simulink model "Full_Integration_with_sensor_redudancy"  (R2024b)
settings: Solver=VariableStepAuto  StartTime=0.0  StopTime=500  RelTol=1e-3
undefined symbols (not defined in the file): Bm1, Bm2, Br, Bsc, Btr, Continuous, G, Im1, Im2, Isw, Jtr, Ke, Ke2, kp, kr, ks, Ksc, Ksr, Kt, Kt2, ktr, Kv1, Kv2, L1, L2, lf, lr, Mr, N, n, n1, R1, R2, rp, Tfrc, Time, to, Vx
libraries: simulink_extras x3, simulink x2, slpidlib x1, ctrlSharedLib x1
settings Model: Creator=Timothy  LastModifiedBy=HP
settings OptimizationCC: ReuseModelBlockBuffer=off
settings RTWCC: GPUComputeCapability=3.5

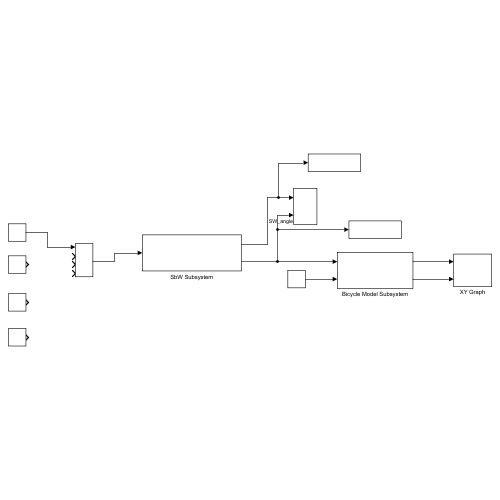
[thumbnail: Simulink's stored preview of the top-level diagram]
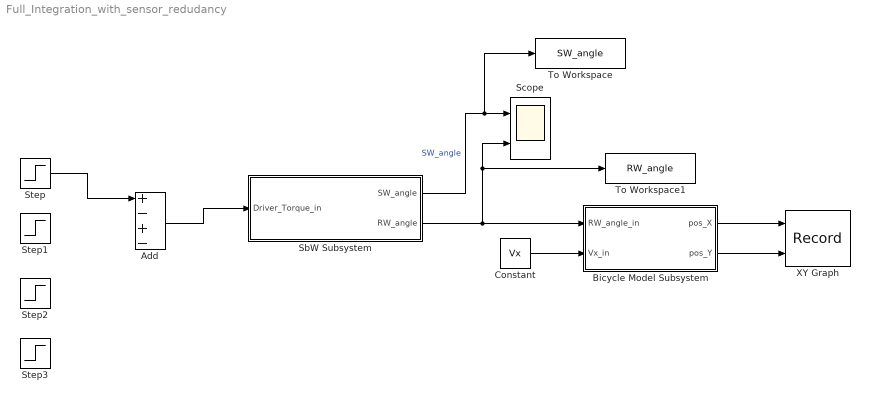
== system Full_Integration_with_sensor_redudancy ==
  Add : Sum  Inputs=+-+-
  Bicycle Model Subsystem : Subsystem
  Constant : Constant  Value=Vx
  SbW Subsystem : Subsystem
  Scope : Scope  NumInputPorts=2
  Step : Step  Time=0  After=0.5  SampleTime=0
  Step1 : Step  Time=30.1  After=0.5  SampleTime=0
  Step2 : Step  Time=60  After=-0.5  SampleTime=0
  Step3 : Step  Time=60.1  After=-0.5  SampleTime=0
  To Workspace : ToWorkspace  VariableName=SW_angle  SaveFormat=Timeseries  SampleTime=-1
  To Workspace1 : ToWorkspace  VariableName=RW_angle  SaveFormat=Timeseries  SampleTime=-1
  XY Graph : Record  FileSettingsInternal="{\"entries\":[{\"content\":{\"excelSettings\":{\"content\":{},\"type\":\"Streamout.ExcelSettings\"}},\"type\":\"Streamout.FileSettingStorage\",\"uuid\":\"\"}],\"packageUris\":[\"http:\\/\\/schema.mathworks.com\\/mf0\\/streamout_blocks\\/R2020a\"],\"version\":\"1.0\"}"  Layout=[1 1]  SignalsInternal="{\"entries\":[{\"content\":{\"signals\":[{\"content\":{\"blockPath\":[],\"dimensions\":[1],\"domain\":\"\",\"lineColor\":\"#a2142f\",\"plots\":[ 1 ],\"port\":1,\"sid\":[\"\"],\"signalID\":1,\"signalName\":\"Bicycle Model Subsystem:1\"},\"type\":\"RecordBlkView.Signal\",\"uuid\":\"\"},{\"content\":{\"blockPath\":[],\"dimensions\":[1],\"domain\":\"\",\"lineColor\":\"#139fff\",\"plots\":[ 1 ],\"port\":2,\"sid\":[\"\"],\"signalID\":2,\"signalName\":\"Bicycle Model Subsystem:2\"},\"type\":\"RecordBlkView.Signal\",\"uuid\":\"\"}]},\"type\":\"RecordBlkView.InputSignals\",\"uuid\":\"\"}],\"packageUris\":[\"http:\\/\\/schema.mathworks.com\\/mf0\\/streamout_blocks\\/R2020a\"],\"version\":\"1.0\"}"  VisualizationBindings="{\"xyplotplugin\":{\"info\":[{\"series\":[{\"bindingParametersList\":[{\"parameter\":\"X-Axis\",\"signalID\":1,\"signalName\":\"Bicycle Model Subsystem:1\"},{\"parameter\":\"Y-Axis\",\"signalID\":2,\"signalName\":\"Bicycle Model Subsystem:2\"}],\"seriesID\":0}],\"subplotID\":1}]}}"  CompatibilityTag=XY
  wires:
  SbW Subsystem/2(RW_angle) -> To Workspace1/1, Scope/2, Bicycle Model Subsystem/1(RW_angle_in)
  SbW Subsystem/1(SW_angle) -> To Workspace/1, Scope/1  "SW_angle"
  Constant/1 -> Bicycle Model Subsystem/2(Vx_in)
  Add/1 -> SbW Subsystem/1(Driver_Torque_in)
  Bicycle Model Subsystem/1(pos_X) -> XY Graph/1
  Bicycle Model Subsystem/2(pos_Y) -> XY Graph/2
  Step/1 -> Add/1

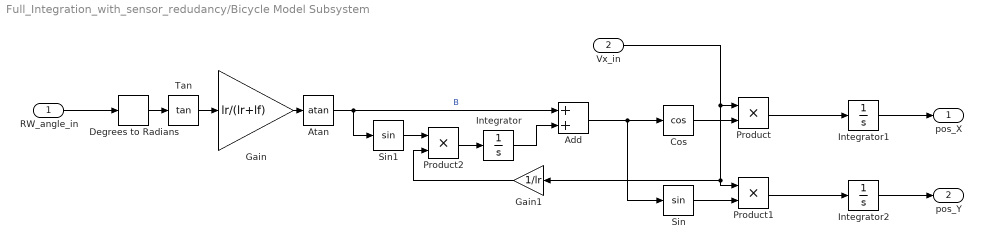
== system Full_Integration_with_sensor_redudancy/Bicycle Model Subsystem ==
  RW_angle_in : Inport
  Vx_in : Inport  Port=2
  Add : Sum
  Atan : Trigonometry  Operator=atan
  Cos : Trigonometry  Operator=cos
  Degrees to Radians : simulink_extras/Transformations/Degrees to Radians
  Gain : Gain  Gain=lr/(lr+lf)
  Gain1 : Gain  Gain=1/lr
  Integrator : Integrator
  Integrator1 : Integrator
  Integrator2 : Integrator
  Product : Product
  Product1 : Product
  Product2 : Product
  Sin : Trigonometry
  Sin1 : Trigonometry
  Tan : Trigonometry  Operator=tan
  pos_X : Outport
  pos_Y : Outport  Port=2
  wires:
  Degrees to Radians/1 -> Tan/1
  Product2/1 -> Integrator/1
  Cos/1 -> Product/2
  Add/1 -> Sin/1, Cos/1
  Atan/1 -> Add/1, Sin1/1  "B"
  Vx_in/1 -> Product1/1, Gain1/1, Product/1
  Integrator1/1 -> pos_X/1
  Gain1/1 -> Product2/2
  Integrator/1 -> Add/2
  Integrator2/1 -> pos_Y/1
  Gain/1 -> Atan/1
  Product/1 -> Integrator1/1
  Product1/1 -> Integrator2/1
  Tan/1 -> Gain/1
  RW_angle_in/1 -> Degrees to Radians/1
  Sin1/1 -> Product2/1
  Sin/1 -> Product1/2

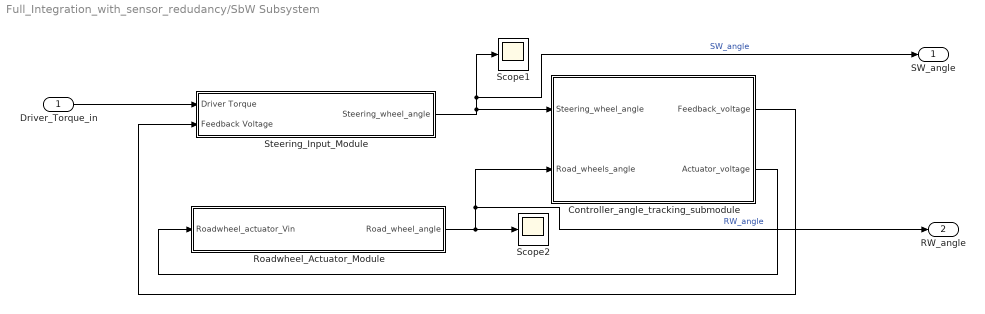
== system Full_Integration_with_sensor_redudancy/SbW Subsystem ==
  Driver_Torque_in : Inport
  Controller_angle_tracking_submodule : Subsystem
  Roadwheel_Actuator_Module : Subsystem
  Scope1 : Scope
  Scope2 : Scope
  Steering_Input_Module : Subsystem
  SW_angle : Outport
  RW_angle : Outport  Port=2
  wires:
  Roadwheel_Actuator_Module/1(Road_wheel_angle) -> Scope2/1, RW_angle/1, Controller_angle_tracking_submodule/2(Road_wheels_angle)  "RW_angle"
  Steering_Input_Module/1(Steering_wheel_angle) -> SW_angle/1, Scope1/1, Controller_angle_tracking_submodule/1(Steering_wheel_angle)  "SW_angle"
  Controller_angle_tracking_submodule/2(Actuator_voltage) -> Roadwheel_Actuator_Module/1(Roadwheel_actuator_Vin)
  Driver_Torque_in/1 -> Steering_Input_Module/1(Driver Torque)
  Controller_angle_tracking_submodule/1(Feedback_voltage) -> Steering_Input_Module/2(Feedback Voltage)

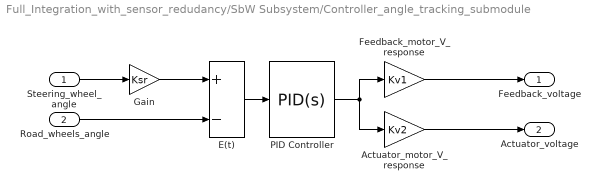
== system Full_Integration_with_sensor_redudancy/SbW Subsystem/Controller_angle_tracking_submodule ==
  Steering_wheel_angle : Inport
  Road_wheels_angle : Inport  Port=2
  Actuator_motor_V_response : Gain  Gain=Kv2
  E(t) : Sum  Inputs=+-
  Feedback_motor_V_response : Gain  Gain=Kv1
  Gain : Gain  Gain=Ksr
  PID Controller : slpidlib/PID Controller  Controller=PID  Form=Parallel  TimeDomain=Continuous-time  UseExternalTs=off  SampleTime=-1  IntegratorMethod=Forward Euler  FilterMethod=Forward Euler  ControllerParametersSource=internal  P=20  I=1  UseKiTs=off  D=-0.5  UseExternalDerivativeSource=off  N=100  UseFilter=on  TunerSelectOption=Transfer Function Based (PID Tuner App)  InitialConditionSource=internal  InitialConditionForIntegrator=0  InitialConditionForFilter=0  DifferentiatorICPrevScaledInput=0  ExternalReset=none  TrackingMode=off  Kt=1  LimitOutput=off  SatLimitsSource=internal  UpperSaturationLimit=100  LowerSaturationLimit=-100  LinearizeAsGain=on  AntiWindupMode=none  Kb=1  LimitIntegrator=off  UpperIntegratorSaturationLimit=inf  LowerIntegratorSaturationLimit=-inf  POutMin=[]  POutMax=[]  IOutMin=[]  IOutMax=[]  DOutMin=[]  DOutMax=[]  NOutMin=[]  NOutMax=[]  SumOutMin=[]  SumOutMax=[]  SaturationOutMin=[]  SaturationOutMax=[]  PParamMin=[]  PParamMax=[]  IParamMin=[]  IParamMax=[]  DParamMin=[]  DParamMax=[]  NParamMin=[]  NParamMax=[]  KbParamMin=[]  KbParamMax=[]  KtParamMin=[]  KtParamMax=[]  KbOutMin=[]  KbOutMax=[]  KtOutMin=[]  KtOutMax=[]  IntegratorOutMin=[]  IntegratorOutMax=[]  FilterOutMin=[]  FilterOutMax=[]  SumI1OutMin=[]  SumI1OutMax=[]  SumI2OutMin=[]  SumI2OutMax=[]  SumI3OutMin=[]  SumI3OutMax=[]  SumI4OutMin=[]  SumI4OutMax=[]  SumDOutMin=[]  SumDOutMax=[]  DifferentiatorOutMin=[]  DifferentiatorOutMax=[]  FilterDiffOutCoefMin=[]  FilterDiffOutCoefMax=[]  ReciprocalOutMin=[]  ReciprocalOutMax=[]  SumDenOutMin=[]  SumDenOutMax=[]  SumNumOutMin=[]  SumNumOutMax=[]  DivideOutMin=[]  DivideOutMax=[]  UdiffTsProdOutMin=[]  UdiffTsProdOutMax=[]  NTsProdOutMin=[]  NTsProdOutMax=[]  UintegralTsProdOutMin=[]  UintegralTsProdOutMax=[]  UngainTsProdOutMin=[]  UngainTsProdOutMax=[]  ClampingZeroOutDataTypeStr=Inherit: Inherit via back propagation  ClampingZeroOutMin=[]  ClampingZeroOutMax=[]  FilterDenConstantOutDataTypeStr=Inherit: Inherit via back propagation  FilterDenConstantOutMin=[]  FilterDenConstantOutMax=[]  PCopyOutDataTypeStr=Inherit: Inherit via back propagation  PCopyOutMin=[]  PCopyOutMax=[]  NCopyOutDataTypeStr=Inherit: Inherit via back propagation  NCopyOutMin=[]  NCopyOutMax=[]  IntegratorContinuousStateAttributes=''  IntegratorStateMustResolveToSignalObject=off  IntegratorRTWStateStorageClass=Auto  FilterContinuousStateAttributes=''  FilterStateMustResolveToSignalObject=off  FilterRTWStateStorageClass=Auto  ParallelPVariant=InternalParameters  IdealPVariant=Disabled  IVariant=InternalParameters  DVariant=InternalParameters  IntegratorVariant=Continuous  SatVariant=Disabled  AWVariant=Passthrough  PCopyVariant=Disabled  TRVariant=Disabled  FdbkBlocksVariant=Forward  IdealPFdbkVariant=Disabled  SatFdbkVariant=Disabled  DerivativeFilterVariant=ContFilter  NVariant=InternalParameters  NCopyVariant=Disabled  FilterICVariant=InternalICsFilter  IntegratorICVariant=InternalICs  ExternalResetVariant=Disabled  TRSumVariant=Passthrough  SumFdbkVariant=Disabled  SumVariant=Sum_PID  TsampFilterVariant=InternalTs  TsampNgainVariant=Passthrough  TsampIntegralVariant=Disabled_SignalSpec  ExternalSaturationOutDataTypeStr=Inherit: Same as second input  DerivativeSourceVariant=ErrorSignal  PreIntVariant=InternalPreInt
  Feedback_voltage : Outport
  Actuator_voltage : Outport  Port=2
  wires:
  Feedback_motor_V_response/1 -> Feedback_voltage/1
  E(t)/1 -> PID Controller/1
  PID Controller/1 -> Actuator_motor_V_response/1, Feedback_motor_V_response/1
  Road_wheels_angle/1 -> E(t)/2
  Steering_wheel_angle/1 -> Gain/1
  Actuator_motor_V_response/1 -> Actuator_voltage/1
  Gain/1 -> E(t)/1

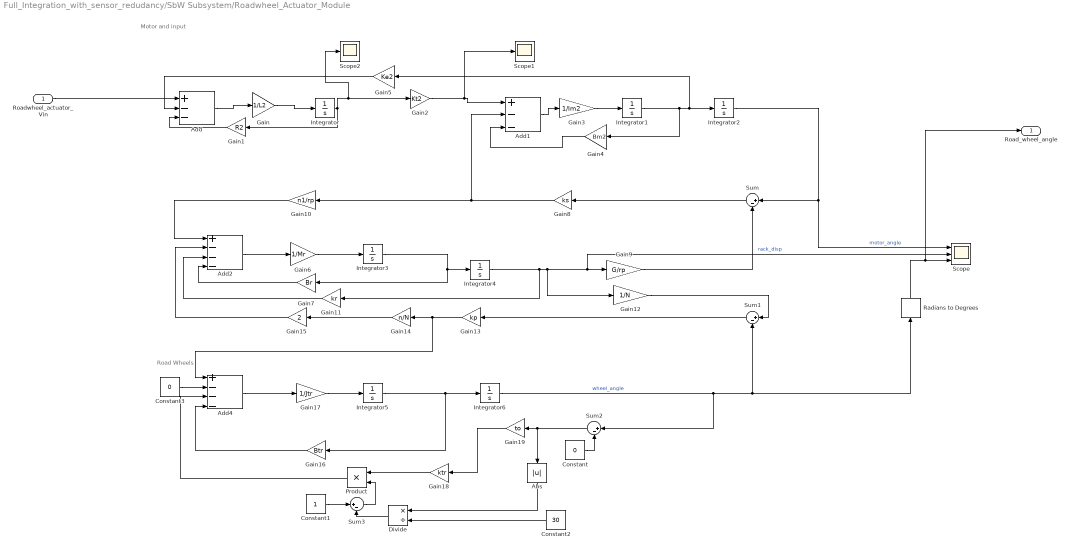
== system Full_Integration_with_sensor_redudancy/SbW Subsystem/Roadwheel_Actuator_Module ==
  note: Road Wheels
  note: Motor and input
  Roadwheel_actuator_Vin : Inport
  Abs : Abs  SaturateOnIntegerOverflow=off
  Add : Sum  Inputs=+--
  Add1 : Sum  Inputs=+--
  Add2 : Sum  Inputs=+---
  Add4 : Sum  Inputs=+---
  Constant : Constant  Value=0
  Constant1 : Constant
  Constant2 : Constant  Value=30
  Constant3 : Constant  Value=0
  Divide : Product  Inputs=*/
  Gain : Gain  Gain=1/L2
  Gain1 : Gain  Gain=R2
  Gain10 : Gain  Gain=n1/rp
  Gain11 : Gain  Gain=kr
  Gain12 : Gain  Gain=1/N
  Gain13 : Gain  Gain=kp
  Gain14 : Gain  Gain=n/N
  Gain15 : Gain  Gain=2
  Gain16 : Gain  Gain=Btr
  Gain17 : Gain  Gain=1/Jtr
  Gain18 : Gain  Gain=ktr
  Gain19 : Gain  Gain=to
  Gain2 : Gain  Gain=Kt2
  Gain3 : Gain  Gain=1/Im2
  Gain4 : Gain  Gain=Bm2
  Gain5 : Gain  Gain=Ke2
  Gain6 : Gain  Gain=1/Mr
  Gain7 : Gain  Gain=Br
  Gain8 : Gain  Gain=ks
  Gain9 : Gain  Gain=G/rp
  Integrator{,1..6} (7 alike) : Integrator
  Product : Product
  Radians to Degrees : simulink_extras/Transformations/Radians to Degrees
  Scope : Scope  NumInputPorts=3
  Scope1 : Scope
  Scope2 : Scope
  Sum{,1..3} (4 alike) : Sum  Inputs=|+-
  Road_wheel_angle : Outport
  wires:
  Gain11/1 -> Add2/3
  Abs/1 -> Divide/1
  Gain5/1 -> Add/2
  Integrator2/1 -> Sum/1, Scope/1  "motor_angle"
  Add1/1 -> Gain3/1
  Gain2/1 -> Scope1/1, Add1/1
  Gain3/1 -> Integrator1/1
  Gain13/1 -> Add4/1, Gain14/1
  Integrator6/1 -> Radians to Degrees/1, Sum1/2, Sum2/1  "wheel_angle"
  Gain6/1 -> Integrator3/1
  Constant1/1 -> Sum3/1
  Roadwheel_actuator_Vin/1 -> Add/1
  Divide/1 -> Sum3/2
  Gain10/1 -> Add2/1
  Integrator/1 -> Gain1/1, Gain2/1, Scope2/1
  Gain1/1 -> Add/3
  Add4/1 -> Gain17/1
  Add/1 -> Gain/1
  Integrator1/1 -> Gain4/1, Gain5/1, Integrator2/1
  Constant2/1 -> Divide/2
  Sum/1 -> Gain8/1
  Sum3/1 -> Product/2
  Gain12/1 -> Sum1/1
  Gain19/1 -> Gain18/1
  Gain15/1 -> Add2/2
  Product/1 -> Add4/3
  Gain18/1 -> Product/1
  Integrator4/1 -> Gain11/1, Gain12/1, Scope/2, Gain9/1  "rack_disp"
  Sum2/1 -> Abs/1, Gain19/1
  Gain9/1 -> Sum/2
  Add2/1 -> Gain6/1
  Integrator3/1 -> Gain7/1, Integrator4/1
  Constant3/1 -> Add4/2
  Gain4/1 -> Add1/3
  Integrator5/1 -> Gain16/1, Integrator6/1
  Gain14/1 -> Gain15/1
  Constant/1 -> Sum2/2
  Sum1/1 -> Gain13/1
  Radians to Degrees/1 -> Road_wheel_angle/1, Scope/3
  Gain16/1 -> Add4/4
  Gain8/1 -> Gain10/1, Add1/2
  Gain17/1 -> Integrator5/1
  Gain/1 -> Integrator/1
  Gain7/1 -> Add2/4

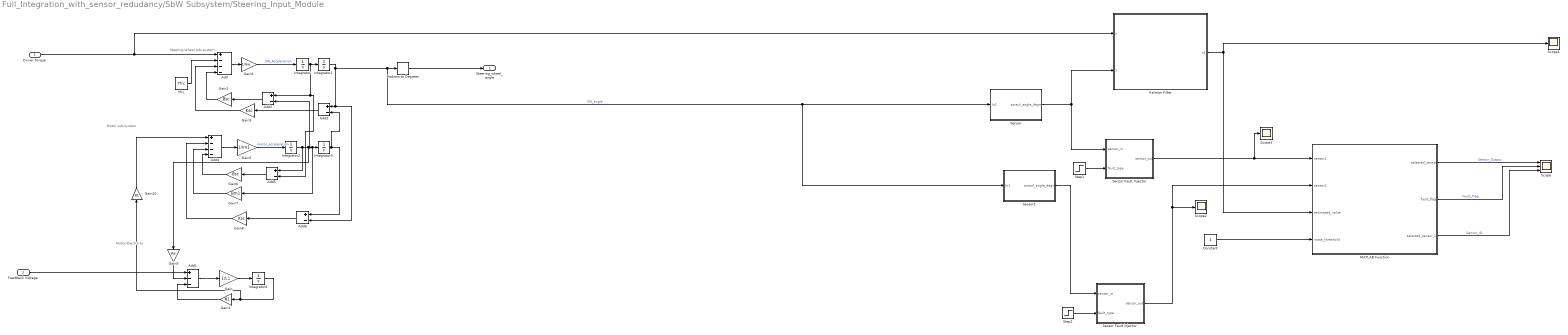
== system Full_Integration_with_sensor_redudancy/SbW Subsystem/Steering_Input_Module ==
  note: Steering Wheel sub-system
  note: Motor-Electrical
  note: Motor sub-system
  Driver Torque : Inport
  Feedback Voltage : Inport  Port=2
  Add : Sum  Inputs=+---
  Add1 : Sum  Inputs=+--
  Add{2..3,5..6} (4 alike) : Sum  Inputs=+-
  Add4 : Sum  Inputs=+---
  Constant : Constant
  Gain : Gain  Gain=1/L1
  Gain1 : Gain  Gain=R1
  Gain10 : Gain  Gain=Kt
  Gain2 : Gain  Gain=Bsc
  Gain3 : Gain  Gain=Ksc
  Gain4 : Gain  Gain=1/Isw
  Gain5 : Gain  Gain=1/Im1
  Gain6 : Gain  Gain=Bsc
  Gain7 : Gain  Gain=Bm1
  Gain8 : Gain  Gain=Ksc
  Gain9 : Gain  Gain=Ke
  Integrator{,1..4} (5 alike) : Integrator
  Kalman Filter : Subsystem
  MATLAB Function : MATLAB Function  TreatAsAtomicUnit=on
  Radians to Degrees : simulink_extras/Transformations/Radians to Degrees
  Scope : Scope  NumInputPorts=3
  Scope1 : Scope
  Scope2 : Scope
  Scope3 : Scope
  Sensor : Subsystem
  Sensor Fault Injector : MATLAB Function  TreatAsAtomicUnit=on
  Sensor Fault injector : MATLAB Function  TreatAsAtomicUnit=on
  Sensor1 : Subsystem
  Step1 : Step  Time=0  SampleTime=0
  Step2 : Step  Time=0  After=2  SampleTime=0
  Tfrc : Constant  Value=Tfrc
  Steering_wheel_angle : Outport
  wires:
  Gain2/1 -> Add/4
  Integrator1/1 -> Add6/2, Add3/1, Sensor1/1(In1), Sensor/1(In1), Radians to Degrees/1  "SW_angle"
  Gain10/1 -> Add4/1
  Gain6/1 -> Add4/4
  Gain8/1 -> Add4/2
  Tfrc/1 -> Add/2
  Gain1/1 -> Add1/3
  Integrator/1 -> Integrator1/1, Add2/1, Add5/2
  Add3/1 -> Gain3/1
  Integrator3/1 -> Add3/2, Add6/1
  Integrator2/1 -> Gain9/1, Add2/2, Gain7/1, Integrator3/1, Add5/1
  Add/1 -> Gain4/1
  Add6/1 -> Gain8/1
  Feedback Voltage/1 -> Add1/1
  Gain/1 -> Integrator4/1
  Gain5/1 -> Integrator2/1  "motor_acceleration"
  Gain7/1 -> Add4/3
  Add1/1 -> Gain/1
  Gain3/1 -> Add/3
  Integrator4/1 -> Gain1/1, Gain10/1
  Add2/1 -> Gain2/1
  Add4/1 -> Gain5/1
  Driver Torque/1 -> Kalman Filter/1(u), Add/1
  Add5/1 -> Gain6/1
  Radians to Degrees/1 -> Steering_wheel_angle/1
  Gain9/1 -> Add1/2
  Gain4/1 -> Integrator/1  "SW_Acceleration"
  Sensor/1(actaul_angle_degre) -> Sensor Fault Injector/1(sensor_in), Kalman Filter/2(y)
  Constant/1 -> MATLAB Function/4(noise_threshold)
  MATLAB Function/1(selected_sensor) -> Scope/1  "Sensor_Output"
  MATLAB Function/2(fault_flag) -> Scope/2  "Fault_Flag"
  MATLAB Function/3(selected_sensor_id) -> Scope/3  "Sensor_ID"
  Kalman Filter/1(s1) -> MATLAB Function/3(estimated_value), Scope1/1
  Sensor1/1(actaul_angle_degre) -> Sensor Fault injector/1(sensor_in)
  Sensor Fault injector/1(sensor_out) -> MATLAB Function/2(sensor2), Scope2/1
  Sensor Fault Injector/1(sensor_out) -> Scope3/1, MATLAB Function/1(sensor1)
  Step1/1 -> Sensor Fault Injector/2(fault_type)
  Step2/1 -> Sensor Fault injector/2(fault_type)

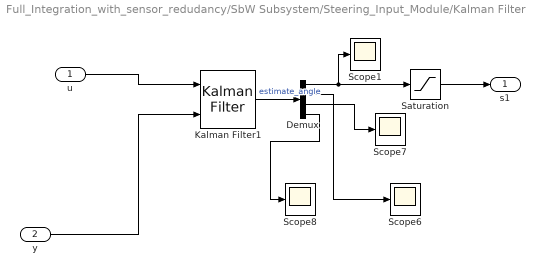
== system Full_Integration_with_sensor_redudancy/SbW Subsystem/Steering_Input_Module/Kalman Filter ==
  u : Inport
  y : Inport  Port=2
  Demux : Demux
  Kalman Filter1 : ctrlSharedLib/Kalman Filter  TimeDomain=Continuous-Time  UseCurrentEstimator=on  ModelSource=Individual A, B, C, D matrices  ModelSourceVariable=sys  A=[0 1 0 0; -(Ksc/Isw) -(Bsc/Isw) (Ksc/Isw) (Bsc/Isw); 0 0 0 1; (Ksc/Im1) (Bsc/Im1) -(Ksc/Im1) -(Bsc+Bm1)/(Im1)]  B=[0; 1/Isw; 0; 1/Im1]  C=[1 0 0 0]  D=0  NumberOfStates=2  NumberOfInputs=2  NumberOfOutputs=2  InitialEstimateSource=Dialog  X0=0  P0=10  UseK=off  UseGH=off  NumberOfProcessNoiseInputs=2  G=1  TimeInvariantG=on  H=0  TimeInvariantH=on  Q="diag([1e-6   1e-4   1e-6   1e-3])"  TimeInvariantQ=on  R=0.0001  TimeInvariantR=on  N=0  TimeInvariantN=on  AddInputPort=on  AddEnablePort=off  OutputEstimatedY=off  OutputP=off  Ts=-1
  Saturation : Saturate  UpperLimit=7.85  LowerLimit=-7.85
  Scope{1,6..8} (4 alike) : Scope
  s1 : Outport
  wires:
  Kalman Filter1/1 -> Demux/1  "estimate_angle"
  Demux/1 -> Scope1/1, Saturation/1
  Demux/2 -> Scope6/1
  y/1 -> Kalman Filter1/2
  u/1 -> Kalman Filter1/1
  Saturation/1 -> s1/1
  Demux/3 -> Scope7/1
  Demux/4 -> Scope8/1

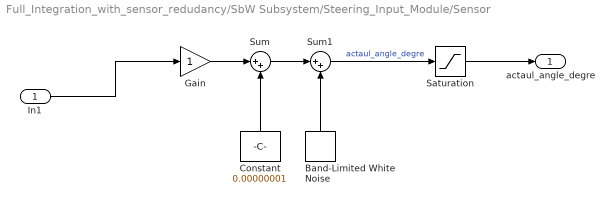
== system Full_Integration_with_sensor_redudancy/SbW Subsystem/Steering_Input_Module/Sensor ==
  In1 : Inport
  Band-Limited White Noise : simulink/Sources/Band-Limited White Noise  Cov=0  Ts=0.01  seed=[23341]
  Constant : Constant  Value=0.00000001  SampleTime=0.01
  Gain : Gain
  Saturation : Saturate  UpperLimit=7.85  LowerLimit=-7.85
  Sum : Sum  Inputs=|++
  Sum1 : Sum  Inputs=|++
  actaul_angle_degre : Outport
  wires:
  Gain/1 -> Sum/1
  Sum/1 -> Sum1/1
  Constant/1 -> Sum/2
  Sum1/1 -> Saturation/1  "actaul_angle_degre"
  In1/1 -> Gain/1
  Band-Limited White Noise/1 -> Sum1/2
  Saturation/1 -> actaul_angle_degre/1

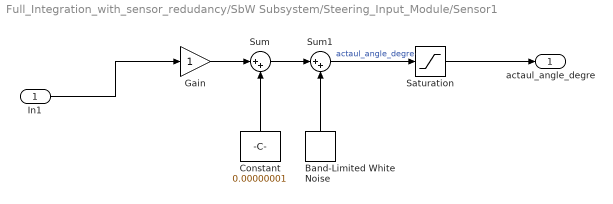
== system Full_Integration_with_sensor_redudancy/SbW Subsystem/Steering_Input_Module/Sensor1 ==
  In1 : Inport
  Band-Limited White Noise : simulink/Sources/Band-Limited White Noise  Cov=0  Ts=1  seed=[23341]
  Constant : Constant  Value=0.00000001  SampleTime=0
  Gain : Gain
  Saturation : Saturate  UpperLimit=7.85  LowerLimit=-7.85
  Sum : Sum  Inputs=|++
  Sum1 : Sum  Inputs=|++
  actaul_angle_degre : Outport
  wires:
  Band-Limited White Noise/1 -> Sum1/2
  In1/1 -> Gain/1
  Sum1/1 -> Saturation/1  "actaul_angle_degre"
  Constant/1 -> Sum/2
  Sum/1 -> Sum1/1
  Gain/1 -> Sum/1
  Saturation/1 -> actaul_angle_degre/1

== matlab function Full_Integration_with_sensor_redudancy/SbW Subsystem/Steering_Input_Module/Sensor Fault Injector ==
  settings: updateMethod=DISCRETE  sampleTime=1
  data: sensor_in input; sensor_out output; fault_type input

function sensor_out = Sensor_fault(sensor_in, fault_type)

% Define fault magnitudes here
bias  = 5.0;          % constant offset added in case 1
noise_std = 3.0;      % noise standard deviation for case 2

% Box-Muller (randn not supported in Simulink MATLAB Function block)
u1 = rand(); u2 = rand();
if u1 < 1e-10; u1 = 1e-10; end
noise = noise_std * sqrt(-2.0 * log(u1)) * cos(2.0 * pi * u2);

switch round(fault_type)
    case 0
        sensor_out = sensor_in;              % Normal
    case 1
        sensor_out = sensor_in + bias;       % Bias
    case 2
        sensor_out = sensor_in + noise;      % Noisy
    case 3
        sensor_out = 0;                      % Short circuit
    otherwise
        sensor_out = sensor_in;
end
end

== matlab function Full_Integration_with_sensor_redudancy/SbW Subsystem/Steering_Input_Module/Sensor Fault injector ==
  settings: updateMethod=DISCRETE  sampleTime=1
  data: sensor_in input; sensor_out output; fault_type input

function sensor_out = Sensor_fault(sensor_in, fault_type)

% Define fault magnitudes here
bias  = 5.0;          % constant offset added in case 1
noise_std = 1;      % noise standard deviation for case 2

% Box-Muller (randn not supported in Simulink MATLAB Function block)
u1 = rand(); u2 = rand();
if u1 < 1e-10; u1 = 1e-10; end
noise = noise_std * sqrt(-2.0 * log(u1)) * cos(2.0 * pi * u2);

switch round(fault_type)
    case 0
        sensor_out = sensor_in;              % Normal
    case 1
        sensor_out = sensor_in + bias;       % Bias
    case 2
        sensor_out = sensor_in + noise;      % Noisy
    case 3
        sensor_out = 0;                      % Short circuit
    otherwise
        sensor_out = sensor_in;
end
end

== matlab function Full_Integration_with_sensor_redudancy/SbW Subsystem/Steering_Input_Module/MATLAB Function ==
  settings: updateMethod=DISCRETE  sampleTime=0.01
  data: selected_sensor output; sensor1 input; fault_flag output; sensor2 input; estimated_value input; noise_threshold input; selected_sensor_id output
function [selected_sensor, fault_flag, selected_sensor_id] = ...
         sensor_fault_stable(sensor1, sensor2, estimated_value, noise_threshold)
% Detects all 3 faults from motor_fault injector:
%   Case 1 - Bias:            mean deviates from estimate
%   Case 2 - Noise:           std exceeds noise_threshold  
%   Case 3 - Short circuit:   signal collapses to near zero

persistent buf1 buf2
persistent fc1 fc2
persistent locked1 locked2

BUFFER_SIZE          = 30;
FAULT_CONFIRMATION   = 20;
RECOVERY_CONFIRMATION = 50;

if isempty(buf1)
    buf1    = zeros(BUFFER_SIZE, 1);
    buf2    = zeros(BUFFER_SIZE, 1);
    fc1     = 0;     fc2     = 0;
    locked1 = false; locked2 = false;
end

% --- Update buffers ---
buf1 = [buf1(2:end); sensor1];
buf2 = [buf2(2:end); sensor2];

% --- Detect fault on each sensor ---
f1 = is_faulty(buf1, estimated_value, noise_threshold);
f2 = is_faulty(buf2, estimated_value, noise_threshold);

% --- Hysteresis lock sensor 1 ---
if ~locked1
    if f1
        fc1 = fc1 + 1;
        if fc1 >= FAULT_CONFIRMATION
            locked1 = true;
            fc1     = 0;
        end
    else
        fc1 = max(fc1 - 1, 0);
    end
else
    % Locked faulty — need sustained healthy readings to recover
    if ~f1
        fc1 = fc1 + 1;
        if fc1 >= RECOVERY_CONFIRMATION
            locked1 = false;
            fc1     = 0;
        end
    else
        fc1 = max(fc1 - 1, 0);
    end
end

% --- Hysteresis lock sensor 2 ---
if ~locked2
    if f2
        fc2 = fc2 + 1;
        if fc2 >= FAULT_CONFIRMATION
            locked2 = true;
            fc2     = 0;
        end
    else
        fc2 = max(fc2 - 1, 0);
    end
else
    if ~f2
        fc2 = fc2 + 1;
        if fc2 >= RECOVERY_CONFIRMATION
            locked2 = false;
            fc2     = 0;
        end
    else
        fc2 = max(fc2 - 1, 0);
    end
end

% --- Selection ---
if locked1 && locked2
    selected_sensor    = estimated_value;
    selected_sensor_id = 0;
    fault_flag         = 1;
elseif locked1 && ~locked2
    selected_sensor    = sensor2;
    selected_sensor_id = 2;
    fault_flag         = 1;
elseif ~locked1 && locked2
    selected_sensor    = sensor1;
    selected_sensor_id = 1;
    fault_flag         = 1;
else
    selected_sensor    = sensor1;
    selected_sensor_id = 1;
    fault_flag         = 0;
end
end


% ================================================================
% LOCAL FUNCTION — checks all 3 fault types from motor_fault
% ================================================================
function result = is_faulty(buf, est, noise_threshold)

result = false;
mn     = mean(buf);
sd     = std(buf);

% ----------------------------------------------------------
% FAULT 2 — NOISE
% std of buffer exceeds noise threshold
% motor_fault case 2 adds large noise to sensor_in
% ----------------------------------------------------------
if sd > noise_threshold
    result = true;
    return
end

% ----------------------------------------------------------
% FAULT 1 — BIAS
% Mean of buffer deviates significantly from estimate
% motor_fault case 1 adds a constant bias offset
% std stays LOW so noise check above won't catch this
% ----------------------------------------------------------
bias_threshold = 3 * noise_threshold;
if abs(mn - est) > bias_threshold
    result = true;
    return
end

% ----------------------------------------------------------
% FAULT 3 — SHORT CIRCUIT
% Signal collapses to near zero regardless of true value
% motor_fault case 3 sets sensor_out = 0
% Mean will be near zero, std will also be near zero
% So we check: is mean suspiciously close to zero
% while estimate says it should be something else?
% ----------------------------------------------------------
short_circuit_threshold = noise_threshold * 0.5;
if abs(mn) < short_circuit_threshold && abs(est) > bias_threshold
    result = true;
    return
end

end
